simulink model "Arm_new_inv_kin"  (R2014b)
settings: Solver=ode45  StartTime=0.0  StopTime=1  RelTol=1e-3
libraries: mblibv1 x29
settings Model: Creator=Qizong  LastModifiedBy=Qizong
settings SimMechanicsCC: VisOnUpdateDiagram=on  VisDuringSimulation=on

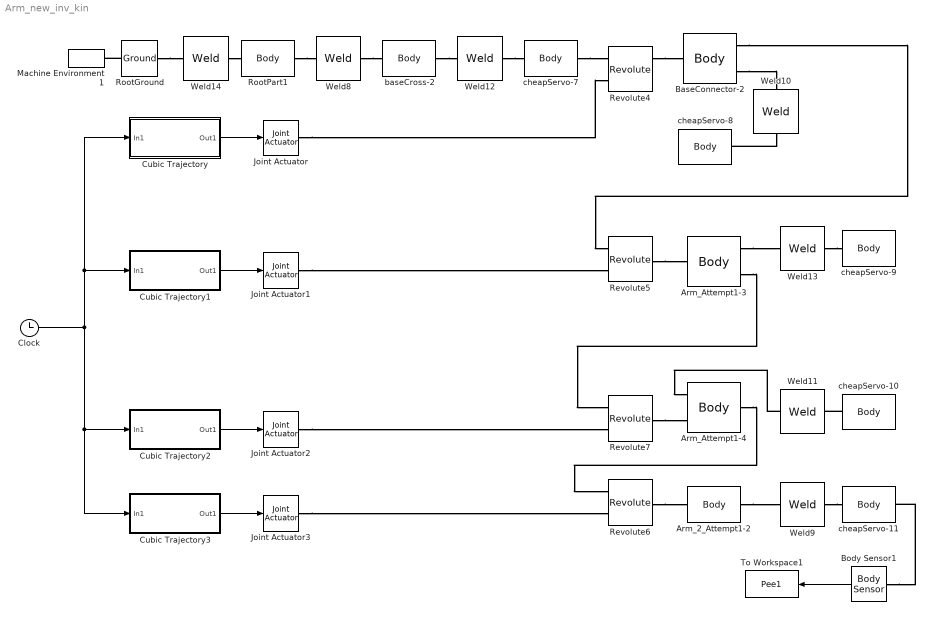
== system Arm_new_inv_kin ==
  Arm_2_Attempt1-2 : mblibv1/Bodies/Body  LConnTagsString=CS3  RConnTagsString=CS2  UpdateFromCAD=on  DialogClass=MechanicalBodyBlock  Mass=0.00482788  MassUnits=kg  InertiaUnits=kg*m^2  Inertia=[1.93456e-06,-1.28538e-09,1.03955e-07;-1.28538e-09,2.88684e-06,-1.81312e-09;1.03955e-07,-1.81312e-09,1.07e-06]  Shape=Cylinder  ShapeDims=[1 1]  ShapeUnits=m  ShapeUse=false  Density=1  DensityUnits=kg/m^3  DensityUse=false  GraphicsMode=GFXFILE  GraphicsFileName=Arm_new - Arm_2_Attempt1-1.STL  BodyColorSelMode=COLORPALETTE  BodyColor=[0.792157;0.819608;0.933333]  AttachedToCS=CS1  CG=Right$CG$[0.0802063 0.117359 0.26392]$WORLD$WORLD$m$[0 0 -1;0 1 0;1 0 0]$3x3 Transform$rad$WORLD$false$none  WorkingFrames=Right$CS1$[0.0387132 0.111386 0.303805]$WORLD$WORLD$m$[0 0 -1;0 1 0;1 0 0]$3x3 Transform$rad$WORLD$false$none#Right$CS2$[0.0387132 0.111386 0.303805]$WORLD$WORLD$m$[1 0 0;0 1 0;0 0 1]$3x3 Transform$rad$WORLD$true$none#Left$CS3$[0.0587132 0.117456 0.279]$WORLD$WORLD$m$[1 0 0;0 1 0;0 0 1]$3x3 Transform$rad$WORLD$true$none  CGPos=[0.0802063 0.117359 0.26392]  CGRot=[0 0 -1;0 1 0;1 0 0]  CS0Pos=[]  CS0Rot=[]  CS1Pos=[0.0387132 0.111386 0.303805]  CS1Rot=[0 0 -1;0 1 0;1 0 0]  CS2Pos=[0.0387132 0.111386 0.303805]  CS2Rot=[1 0 0;0 1 0;0 0 1]  CS3Pos=[0.0587132 0.117456 0.279]  CS3Rot=[1 0 0;0 1 0;0 0 1]  CS4Pos=[]  CS4Rot=[]  CS5Pos=[]  CS5Rot=[]  CS6Pos=[]  CS6Rot=[]  CS7Pos=[]  CS7Rot=[]  CS8Pos=[]  CS8Rot=[]  CS9Pos=[]  CS9Rot=[]  CS10Pos=[]  CS10Rot=[]  CS11Pos=[]  CS11Rot=[]  CS12Pos=[]  CS12Rot=[]  CS13Pos=[]  CS13Rot=[]  CS14Pos=[]  CS14Rot=[]  CS15Pos=[]  CS15Rot=[]  CS16Pos=[]  CS16Rot=[]  CS17Pos=[]  CS17Rot=[]  CS18Pos=[]  CS18Rot=[]  CS19Pos=[]  CS19Rot=[]  CS20Pos=[]  CS20Rot=[]
  Arm_Attempt1-3 : mblibv1/Bodies/Body  LConnTagsString=CS2  RConnTagsString=CS3|CS4  UpdateFromCAD=on  DialogClass=MechanicalBodyBlock  Mass=0.00663008  MassUnits=kg  InertiaUnits=kg*m^2  Inertia=[3.57587e-06,1.12045e-09,4.59326e-07;1.12045e-09,4.47292e-06,-5.09042e-09;4.59326e-07,-5.09042e-09,1.05685e-06]  Shape=Cylinder  ShapeDims=[1 1]  ShapeUnits=m  ShapeUse=false  Density=1  DensityUnits=kg/m^3  DensityUse=false  GraphicsMode=GFXFILE  GraphicsFileName=Arm_new - Arm_Attempt1-1.STL  BodyColorSelMode=COLORPALETTE  BodyColor=[0.792157;0.819608;0.933333]  AttachedToCS=CS1  CG=Right$CG$[0.0109911 0.0413075 0.267024]$WORLD$WORLD$m$[0 -1 0;0 0 -1;1 0 0]$3x3 Transform$rad$WORLD$false$none  WorkingFrames=Right$CS1$[0.0169693 -0.00863884 0.305399]$WORLD$WORLD$m$[0 -1 0;0 0 -1;1 0 0]$3x3 Transform$rad$WORLD$false$none#Left$CS2$[0.0108991 0.00236116 0.279]$WORLD$WORLD$m$[1 0 0;0 1 0;0 0 1]$3x3 Transform$rad$WORLD$true$none#Right$CS3$[0.00496925 0.0753612 0.277464]$WORLD$WORLD$m$[1 0 0;0 1 0;0 0 1]$3x3 Transform$rad$WORLD$true$none#Right$CS4$[0.0109693 0.0698112 0.279]$WORLD$WORLD$m$[1 0 0;0 1 0;0 0 1]$3x3 Transform$rad$WORLD$true$none  CGPos=[0.0109911 0.0413075 0.267024]  CGRot=[0 -1 0;0 0 -1;1 0 0]  CS0Pos=[]  CS0Rot=[]  CS1Pos=[0.0169693 -0.00863884 0.305399]  CS1Rot=[0 -1 0;0 0 -1;1 0 0]  CS2Pos=[0.0108991 0.00236116 0.279]  CS2Rot=[1 0 0;0 1 0;0 0 1]  CS3Pos=[0.00496925 0.0753612 0.277464]  CS3Rot=[1 0 0;0 1 0;0 0 1]  CS4Pos=[0.0109693 0.0698112 0.279]  CS4Rot=[1 0 0;0 1 0;0 0 1]  CS5Pos=[]  CS5Rot=[]  CS6Pos=[]  CS6Rot=[]  CS7Pos=[]  CS7Rot=[]  CS8Pos=[]  CS8Rot=[]  CS9Pos=[]  CS9Rot=[]  CS10Pos=[]  CS10Rot=[]  CS11Pos=[]  CS11Rot=[]  CS12Pos=[]  CS12Rot=[]  CS13Pos=[]  CS13Rot=[]  CS14Pos=[]  CS14Rot=[]  CS15Pos=[]  CS15Rot=[]  CS16Pos=[]  CS16Rot=[]  CS17Pos=[]  CS17Rot=[]  CS18Pos=[]  CS18Rot=[]  CS19Pos=[]  CS19Rot=[]  CS20Pos=[]  CS20Rot=[]
  Arm_Attempt1-4 : mblibv1/Bodies/Body  LConnTagsString=CS2|CS4  RConnTagsString=CS3  UpdateFromCAD=on  DialogClass=MechanicalBodyBlock  Mass=0.00663008  MassUnits=kg  InertiaUnits=kg*m^2  Inertia=[3.57587e-06,1.12045e-09,4.59326e-07;1.12045e-09,4.47292e-06,-5.09042e-09;4.59326e-07,-5.09042e-09,1.05685e-06]  Shape=Cylinder  ShapeDims=[1 1]  ShapeUnits=m  ShapeUse=false  Density=1  DensityUnits=kg/m^3  DensityUse=false  GraphicsMode=GFXFILE  GraphicsFileName=Arm_new - Arm_Attempt1-2.STL  BodyColorSelMode=COLORPALETTE  BodyColor=[0.792157;0.819608;0.933333]  AttachedToCS=CS1  CG=Right$CG$[0.0385735 0.0972853 0.267024]$WORLD$WORLD$m$[0 -0.707107 -0.707107;0 0.707107 -0.707107;1 0 0]$3x3 Transform$rad$WORLD$false$none  WorkingFrames=Right$CS1$[0.00748332 0.0577407 0.305399]$WORLD$WORLD$m$[0 -0.707107 -0.707107;0 0.707107 -0.707107;1 0 0]$3x3 Transform$rad$WORLD$false$none#Left$CS2$[0.0667389 0.117279 0.265014]$WORLD$WORLD$m$[1 0 0;0 1 0;0 0 1]$3x3 Transform$rad$WORLD$true$none#Right$CS3$[0.0587132 0.117456 0.279]$WORLD$WORLD$m$[1 0 0;0 1 0;0 0 1]$3x3 Transform$rad$WORLD$true$none#Left$CS4$[0.0109693 0.0698112 0.279]$WORLD$WORLD$m$[1 0 0;0 1 0;0 0 1]$3x3 Transform$rad$WORLD$true$none  CGPos=[0.0385735 0.0972853 0.267024]  CGRot=[0 -0.707107 -0.707107;0 0.707107 -0.707107;1 0 0]  CS0Pos=[]  CS0Rot=[]  CS1Pos=[0.00748332 0.0577407 0.305399]  CS1Rot=[0 -0.707107 -0.707107;0 0.707107 -0.707107;1 0 0]  CS2Pos=[0.0667389 0.117279 0.265014]  CS2Rot=[1 0 0;0 1 0;0 0 1]  CS3Pos=[0.0587132 0.117456 0.279]  CS3Rot=[1 0 0;0 1 0;0 0 1]  CS4Pos=[0.0109693 0.0698112 0.279]  CS4Rot=[1 0 0;0 1 0;0 0 1]  CS5Pos=[]  CS5Rot=[]  CS6Pos=[]  CS6Rot=[]  CS7Pos=[]  CS7Rot=[]  CS8Pos=[]  CS8Rot=[]  CS9Pos=[]  CS9Rot=[]  CS10Pos=[]  CS10Rot=[]  CS11Pos=[]  CS11Rot=[]  CS12Pos=[]  CS12Rot=[]  CS13Pos=[]  CS13Rot=[]  CS14Pos=[]  CS14Rot=[]  CS15Pos=[]  CS15Rot=[]  CS16Pos=[]  CS16Rot=[]  CS17Pos=[]  CS17Rot=[]  CS18Pos=[]  CS18Rot=[]  CS19Pos=[]  CS19Rot=[]  CS20Pos=[]  CS20Rot=[]
  BaseConnector-2 : mblibv1/Bodies/Body  LConnTagsString=CS2  RConnTagsString=CS3|CS4  UpdateFromCAD=on  DialogClass=MechanicalBodyBlock  Mass=0.00289161  MassUnits=kg  InertiaUnits=kg*m^2  Inertia=[1.81369e-07,-9.46923e-10,-2.62761e-09;-9.46923e-10,3.3813e-07,-2.11475e-08;-2.62761e-09,-2.11475e-08,2.75643e-07]  Shape=Cylinder  ShapeDims=[1 1]  ShapeUnits=m  ShapeUse=false  Density=1  DensityUnits=kg/m^3  DensityUse=false  GraphicsMode=GFXFILE  GraphicsFileName=Arm_new - BaseConnector-1.STL  BodyColorSelMode=COLORPALETTE  BodyColor=[1;1;1]  AttachedToCS=CS1  CG=Right$CG$[0.00564211 -0.00116004 0.271229]$WORLD$WORLD$m$[1 0 0;0 1 0;0 0 1]$3x3 Transform$rad$WORLD$false$none  WorkingFrames=Right$CS1$[0.00554911 -0.00353884 0.2601]$WORLD$WORLD$m$[1 0 0;0 1 0;0 0 1]$3x3 Transform$rad$WORLD$false$none#Left$CS2$[0.00554911 -0.00353884 0.27]$WORLD$WORLD$m$[1 0 0;0 1 0;0 0 1]$3x3 Transform$rad$WORLD$true$none#Right$CS3$[0.0108991 0.00236116 0.279]$WORLD$WORLD$m$[1 0 0;0 1 0;0 0 1]$3x3 Transform$rad$WORLD$true$none#Right$CS4$[0.00554911 -0.00353884 0.2601]$WORLD$WORLD$m$[1 0 0;0 1 0;0 0 1]$3x3 Transform$rad$WORLD$true$none  CGPos=[0.00564211 -0.00116004 0.271229]  CGRot=[1 0 0;0 1 0;0 0 1]  CS0Pos=[]  CS0Rot=[]  CS1Pos=[0.00554911 -0.00353884 0.2601]  CS1Rot=[1 0 0;0 1 0;0 0 1]  CS2Pos=[0.00554911 -0.00353884 0.27]  CS2Rot=[1 0 0;0 1 0;0 0 1]  CS3Pos=[0.0108991 0.00236116 0.279]  CS3Rot=[1 0 0;0 1 0;0 0 1]  CS4Pos=[0.00554911 -0.00353884 0.2601]  CS4Rot=[1 0 0;0 1 0;0 0 1]  CS5Pos=[]  CS5Rot=[]  CS6Pos=[]  CS6Rot=[]  CS7Pos=[]  CS7Rot=[]  CS8Pos=[]  CS8Rot=[]  CS9Pos=[]  CS9Rot=[]  CS10Pos=[]  CS10Rot=[]  CS11Pos=[]  CS11Rot=[]  CS12Pos=[]  CS12Rot=[]  CS13Pos=[]  CS13Rot=[]  CS14Pos=[]  CS14Rot=[]  CS15Pos=[]  CS15Rot=[]  CS16Pos=[]  CS16Rot=[]  CS17Pos=[]  CS17Rot=[]  CS18Pos=[]  CS18Rot=[]  CS19Pos=[]  CS19Rot=[]  CS20Pos=[]  CS20Rot=[]
  Body Sensor1 : mblibv1/Sensors &  Actuators/Body Sensor  UpdateFromCAD=off  PhysicalDomain=Mechanical  PortType=blob  Muxed=on  Pose=off  Angle=on  AngleUnits=deg  ArcVelocity=off  ArcVelocityUnits=deg/s  ArcAcceleration=off  ArcAccelerationUnits=deg/s^2  CoordPosition=on  CoordPositionUnits=m  Velocity=off  VelocityUnits=m/s  Acceleration=off  AccelerationUnits=m/s^2  Quaternion=on  QuaternionDT=off  QuaternionDDT=off  QuaternionUnits=off  OutputVector=[1]  ActiveIO=on  Width=3  DialogClass=MechanicalSensorBlock  ReferenceFrame=Absolute (World)
  Clock : Clock
  Cubic Trajectory : Subsystem  mask(Cubic Trajectory){}
  Cubic Trajectory1 : Subsystem  mask(Cubic Trajectory){}
  Cubic Trajectory2 : Subsystem  mask(Cubic Trajectory){}
  Cubic Trajectory3 : Subsystem  mask(Cubic Trajectory){}
  Joint Actuator{,1..3} (4 alike) : mblibv1/Sensors &  Actuators/Joint Actuator  UpdateFromCAD=off  PhysicalDomain=Mechanical  PortType=blob  ActuationStyle=Motion  AngleUnits=rad  ArcVelocityUnits=rad/s  ArcAccelerationUnits=rad/s^2  CoordPositionUnits=m  VelocityUnits=m/s  AccelerationUnits=m/s^2  ForceUnits=N  TorqueUnits=N*m  ActiveIO=on  Width=3  DialogClass=MechanicalActuatorBlock  Primitive=R1  ReferenceFrame=Absolute (World)
  Machine Environment1 : mblibv1/Bodies/Machine Environment  PortType=env  PhysicalDomain=Mechanical  DialogTemplateClass=MECH.MachineEnvironment  SyncWhenCopied=off  Gravity=[0 -9.81 0]  GravityUnits=m/s^2  GravityAsSignal=off  Dimensionality=Auto-detect  AnalysisType=Forward dynamics  LinearAssemblyTolerance=1e-3  LinearAssemblyToleranceUnits=m  AngularAssemblyTolerance=1e-3  AngularAssemblyToleranceUnits=rad  ConstraintSolverType=Stabilizing  ConstraintRelTolerance=1e-4  ConstraintAbsTolerance=1e-4  UseRobustSingularityHandling=off  RedundancyAnalysisToleranceType=Automatically select tolerance  RedundancyAnalysisTolerance=1e-14  StatePerturbationType=Fixed  PerturbationSize=1e-5  VisualizeMachine=on  BodyVisualizationType=Use model default body geometries  BodyColorSelMode=Use model default  DefaultBodyColor=[1 0 0]
  Revolute4 : mblibv1/Joints/Revolute  LConnTagsString=__newl0|SA1  RConnTagsString=__newr0|SA1  UpdateFromCAD=on  NumSAPorts=2  CutJoint=off  MarkAsCut=off  Primitives=prismatic  PrimitiveProps=R1$World$[0,1,0]$revolute  DialogClass=JointBlock  R1Axis=[0,1,0]
  Revolute5 : mblibv1/Joints/Revolute  LConnTagsString=__newl0|SA1  RConnTagsString=__newr0  UpdateFromCAD=on  NumSAPorts=1  CutJoint=off  MarkAsCut=off  Primitives=prismatic  PrimitiveProps=R1$World$[0,0,-1]$revolute  DialogClass=JointBlock  R1Axis=[0,0,-1]
  Revolute6 : mblibv1/Joints/Revolute  LConnTagsString=__newl0|SA1  RConnTagsString=__newr0  UpdateFromCAD=on  NumSAPorts=1  CutJoint=off  MarkAsCut=off  Primitives=prismatic  PrimitiveProps=R1$World$[0,0,-1]$revolute  DialogClass=JointBlock  R1Axis=[0,0,-1]
  Revolute7 : mblibv1/Joints/Revolute  LConnTagsString=__newl0|SA1  RConnTagsString=__newr0  UpdateFromCAD=on  NumSAPorts=1  CutJoint=off  MarkAsCut=off  Primitives=prismatic  PrimitiveProps=R1$World$[0,0,-1]$revolute  DialogClass=JointBlock  R1Axis=[0,0,-1]
  RootGround : mblibv1/Bodies/Ground  UpdateFromCAD=on  LeftPortType=env  RightPortType=workingframe  PhysicalDomain=Mechanical  DialogClass=GroundBlock  CoordPosition=[0.024952,0.026403,0.267905]  CoordPositionUnits=m  StateVectorMgrId=2  MachineId=[1 0]  ShowEnvPort=on  ParameterChecksum=[449264359, 1693856497, 1829625602, 1228565225]  TopologyChecksum=[1919634279, 3543996490, 3153834687, 3124392432]
  RootPart1 : mblibv1/Bodies/Body  LConnTagsString=CS3  RConnTagsString=CS2  UpdateFromCAD=on  DialogClass=MechanicalBodyBlock  Mass=0  MassUnits=kg  InertiaUnits=kg*m^2  Inertia=[0,0,0;0,0,0;0,0,0]  Shape=Cylinder  ShapeDims=[1 1]  ShapeUnits=m  ShapeUse=false  Density=1  DensityUnits=kg/m^3  DensityUse=false  GraphicsMode=MACHINE_DEFAULT  BodyColorSelMode=MACHINE_DEFAULT  BodyColor=[1;0;0]  AttachedToCS=CS1  CG=Right$CG$[0.024952 0.026403 0.267905]$WORLD$WORLD$m$[1 0 0;0 1 0;0 0 1]$3x3 Transform$rad$WORLD$false$none  WorkingFrames=Right$CS1$[0 0 0]$WORLD$WORLD$m$[1 0 0;0 1 0;0 0 1]$3x3 Transform$rad$WORLD$false$none#Right$CS2$[0.00554913 -0.0339934 0.27051]$WORLD$WORLD$m$[1 0 0;0 1 0;0 0 1]$3x3 Transform$rad$WORLD$true$none#Left$CS3$[0.024952 0.026403 0.267905]$WORLD$WORLD$m$[1 0 0;0 1 0;0 0 1]$3x3 Transform$rad$WORLD$true$none  CGPos=[0.024952 0.026403 0.267905]  CGRot=[1 0 0;0 1 0;0 0 1]  CS0Pos=[]  CS0Rot=[]  CS1Pos=[0 0 0]  CS1Rot=[1 0 0;0 1 0;0 0 1]  CS2Pos=[0.00554913 -0.0339934 0.27051]  CS2Rot=[1 0 0;0 1 0;0 0 1]  CS3Pos=[0.024952 0.026403 0.267905]  CS3Rot=[1 0 0;0 1 0;0 0 1]  CS4Pos=[]  CS4Rot=[]  CS5Pos=[]  CS5Rot=[]  CS6Pos=[]  CS6Rot=[]  CS7Pos=[]  CS7Rot=[]  CS8Pos=[]  CS8Rot=[]  CS9Pos=[]  CS9Rot=[]  CS10Pos=[]  CS10Rot=[]  CS11Pos=[]  CS11Rot=[]  CS12Pos=[]  CS12Rot=[]  CS13Pos=[]  CS13Rot=[]  CS14Pos=[]  CS14Rot=[]  CS15Pos=[]  CS15Rot=[]  CS16Pos=[]  CS16Rot=[]  CS17Pos=[]  CS17Rot=[]  CS18Pos=[]  CS18Rot=[]  CS19Pos=[]  CS19Rot=[]  CS20Pos=[]  CS20Rot=[]
  To Workspace1 : ToWorkspace  VariableName=Pee1  SaveFormat=Timeseries  SampleTime=-1
  Weld{8..14} (7 alike) : mblibv1/Joints/Weld  LConnTagsString=__newl0  RConnTagsString=__newr0  UpdateFromCAD=on  NumSAPorts=0  CutJoint=off  MarkAsCut=off  Primitives=weld  PrimitiveProps=W$WORLD$[0.57735,0.57735,0.57735]$weld  DialogClass=JointBlock  WAxis=[0.57735,0.57735,0.57735]
  baseCross-2 : mblibv1/Bodies/Body  LConnTagsString=CS2  RConnTagsString=CS3  UpdateFromCAD=on  DialogClass=MechanicalBodyBlock  Mass=0.0338588  MassUnits=kg  InertiaUnits=kg*m^2  Inertia=[9.50419e-05,-4.72341e-14,1.07796e-10;-4.72341e-14,0.000189164,-1.55231e-07;1.07796e-10,-1.55231e-07,9.48987e-05]  Shape=Cylinder  ShapeDims=[1 1]  ShapeUnits=m  ShapeUse=false  Density=1  DensityUnits=kg/m^3  DensityUse=false  GraphicsMode=GFXFILE  GraphicsFileName=Arm_new - baseCross-1.STL  BodyColorSelMode=COLORPALETTE  BodyColor=[1;1;1]  AttachedToCS=CS1  CG=Right$CG$[0.00554913 -0.0339934 0.27051]$WORLD$WORLD$m$[1 0 0;0 1 0;0 0 1]$3x3 Transform$rad$WORLD$false$none  WorkingFrames=Right$CS1$[0.00554911 -0.0334388 0.27]$WORLD$WORLD$m$[1 0 0;0 1 0;0 0 1]$3x3 Transform$rad$WORLD$false$none#Left$CS2$[0.00554913 -0.0339934 0.27051]$WORLD$WORLD$m$[1 0 0;0 1 0;0 0 1]$3x3 Transform$rad$WORLD$true$none#Right$CS3$[-0.000350892 -0.0175388 0.27]$WORLD$WORLD$m$[1 0 0;0 1 0;0 0 1]$3x3 Transform$rad$WORLD$true$none  CGPos=[0.00554913 -0.0339934 0.27051]  CGRot=[1 0 0;0 1 0;0 0 1]  CS0Pos=[]  CS0Rot=[]  CS1Pos=[0.00554911 -0.0334388 0.27]  CS1Rot=[1 0 0;0 1 0;0 0 1]  CS2Pos=[0.00554913 -0.0339934 0.27051]  CS2Rot=[1 0 0;0 1 0;0 0 1]  CS3Pos=[-0.000350892 -0.0175388 0.27]  CS3Rot=[1 0 0;0 1 0;0 0 1]  CS4Pos=[]  CS4Rot=[]  CS5Pos=[]  CS5Rot=[]  CS6Pos=[]  CS6Rot=[]  CS7Pos=[]  CS7Rot=[]  CS8Pos=[]  CS8Rot=[]  CS9Pos=[]  CS9Rot=[]  CS10Pos=[]  CS10Rot=[]  CS11Pos=[]  CS11Rot=[]  CS12Pos=[]  CS12Rot=[]  CS13Pos=[]  CS13Rot=[]  CS14Pos=[]  CS14Rot=[]  CS15Pos=[]  CS15Rot=[]  CS16Pos=[]  CS16Rot=[]  CS17Pos=[]  CS17Rot=[]  CS18Pos=[]  CS18Rot=[]  CS19Pos=[]  CS19Rot=[]  CS20Pos=[]  CS20Rot=[]
  cheapServo-10 : mblibv1/Bodies/Body  RConnTagsString=CS2  UpdateFromCAD=on  DialogClass=MechanicalBodyBlock  Mass=0.00769542  MassUnits=kg  InertiaUnits=kg*m^2  Inertia=[4.96531e-07,3.23519e-08,0;3.23519e-08,4.44048e-07,0;0,0,7.67618e-07]  Shape=Cylinder  ShapeDims=[1 1]  ShapeUnits=m  ShapeUse=false  Density=1  DensityUnits=kg/m^3  DensityUse=false  GraphicsMode=GFXFILE  GraphicsFileName=Arm_new - cheapServo-5.STL  BodyColorSelMode=COLORPALETTE  BodyColor=[0.494118;0.494118;0.494118]  AttachedToCS=CS1  CG=Right$CG$[0.0548517 0.113736 0.263624]$WORLD$WORLD$m$[-0.707107 0 0.707107;-0.707107 0 -0.707107;0 -1 0]$3x3 Transform$rad$WORLD$false$none  WorkingFrames=Right$CS1$[0.054612 0.113496 0.265014]$WORLD$WORLD$m$[-0.707107 0 0.707107;-0.707107 0 -0.707107;0 -1 0]$3x3 Transform$rad$WORLD$false$none#Right$CS2$[0.0667389 0.117279 0.265014]$WORLD$WORLD$m$[1 0 0;0 1 0;0 0 1]$3x3 Transform$rad$WORLD$true$none  CGPos=[0.0548517 0.113736 0.263624]  CGRot=[-0.707107 0 0.707107;-0.707107 0 -0.707107;0 -1 0]  CS0Pos=[]  CS0Rot=[]  CS1Pos=[0.054612 0.113496 0.265014]  CS1Rot=[-0.707107 0 0.707107;-0.707107 0 -0.707107;0 -1 0]  CS2Pos=[0.0667389 0.117279 0.265014]  CS2Rot=[1 0 0;0 1 0;0 0 1]  CS3Pos=[]  CS3Rot=[]  CS4Pos=[]  CS4Rot=[]  CS5Pos=[]  CS5Rot=[]  CS6Pos=[]  CS6Rot=[]  CS7Pos=[]  CS7Rot=[]  CS8Pos=[]  CS8Rot=[]  CS9Pos=[]  CS9Rot=[]  CS10Pos=[]  CS10Rot=[]  CS11Pos=[]  CS11Rot=[]  CS12Pos=[]  CS12Rot=[]  CS13Pos=[]  CS13Rot=[]  CS14Pos=[]  CS14Rot=[]  CS15Pos=[]  CS15Rot=[]  CS16Pos=[]  CS16Rot=[]  CS17Pos=[]  CS17Rot=[]  CS18Pos=[]  CS18Rot=[]  CS19Pos=[]  CS19Rot=[]  CS20Pos=[]  CS20Rot=[]
  cheapServo-11 : mblibv1/Bodies/Body  LConnTagsString=CS2  RConnTagsString=CS1  UpdateFromCAD=on  DialogClass=MechanicalBodyBlock  Mass=0.00769542  MassUnits=kg  InertiaUnits=kg*m^2  Inertia=[4.96531e-07,3.23519e-08,0;3.23519e-08,4.44048e-07,0;0,0,7.67618e-07]  Shape=Cylinder  ShapeDims=[1 1]  ShapeUnits=m  ShapeUse=false  Density=1  DensityUnits=kg/m^3  DensityUse=false  GraphicsMode=GFXFILE  GraphicsFileName=Arm_new - cheapServo-6.STL  BodyColorSelMode=COLORPALETTE  BodyColor=[0.49412 0.49412 0.49412]  AttachedToCS=CS1  CG=Right$CG$[0.105855 0.117286 0.265314]$WORLD$WORLD$m$[0 1 0;0 0 1;1 0 0]$3x3 Transform$rad$WORLD$false$none  WorkingFrames=Right$CS1$[0.104465 0.117286 0.265653]$World$World$m$[0 1 0;0 0 1;1 0 0]$3x3 Transform$rad$WORLD$true$none#Left$CS2$[0.0387132 0.111386 0.303805]$WORLD$WORLD$m$[1 0 0;0 1 0;0 0 1]$3x3 Transform$rad$WORLD$true$none  CGPos=[0.105855 0.117286 0.265314]  CGRot=[0 1 0;0 0 1;1 0 0]  CS0Pos=[]  CS0Rot=[]  CS1Pos=[0.104465 0.117286 0.265653]  CS1Rot=[0 1 0;0 0 1;1 0 0]  CS2Pos=[0.0387132 0.111386 0.303805]  CS2Rot=[1 0 0;0 1 0;0 0 1]  CS3Pos=[]  CS3Rot=[]  CS4Pos=[]  CS4Rot=[]  CS5Pos=[]  CS5Rot=[]  CS6Pos=[]  CS6Rot=[]  CS7Pos=[]  CS7Rot=[]  CS8Pos=[]  CS8Rot=[]  CS9Pos=[]  CS9Rot=[]  CS10Pos=[]  CS10Rot=[]  CS11Pos=[]  CS11Rot=[]  CS12Pos=[]  CS12Rot=[]  CS13Pos=[]  CS13Rot=[]  CS14Pos=[]  CS14Rot=[]  CS15Pos=[]  CS15Rot=[]  CS16Pos=[]  CS16Rot=[]  CS17Pos=[]  CS17Rot=[]  CS18Pos=[]  CS18Rot=[]  CS19Pos=[]  CS19Rot=[]  CS20Pos=[]  CS20Rot=[]
  cheapServo-7 : mblibv1/Bodies/Body  LConnTagsString=CS3  RConnTagsString=CS2  UpdateFromCAD=on  DialogClass=MechanicalBodyBlock  Mass=0.00769542  MassUnits=kg  InertiaUnits=kg*m^2  Inertia=[4.96531e-07,3.23519e-08,0;3.23519e-08,4.44048e-07,0;0,0,7.67618e-07]  Shape=Cylinder  ShapeDims=[1 1]  ShapeUnits=m  ShapeUse=false  Density=1  DensityUnits=kg/m^3  DensityUse=false  GraphicsMode=GFXFILE  GraphicsFileName=Arm_new - cheapServo-1.STL  BodyColorSelMode=COLORPALETTE  BodyColor=[0.494118;0.494118;0.494118]  AttachedToCS=CS1  CG=Right$CG$[0.00554911 -0.0206986 0.275011]$WORLD$WORLD$m$[0 0 -1;0 1 0;1 0 0]$3x3 Transform$rad$WORLD$false$none  WorkingFrames=Right$CS1$[0.00554911 -0.0220888 0.27535]$WORLD$WORLD$m$[0 0 -1;0 1 0;1 0 0]$3x3 Transform$rad$WORLD$false$none#Right$CS2$[0.00554911 -0.00353884 0.27]$WORLD$WORLD$m$[1 0 0;0 1 0;0 0 1]$3x3 Transform$rad$WORLD$true$none#Left$CS3$[-0.000350892 -0.0175388 0.27]$WORLD$WORLD$m$[1 0 0;0 1 0;0 0 1]$3x3 Transform$rad$WORLD$true$none  CGPos=[0.00554911 -0.0206986 0.275011]  CGRot=[0 0 -1;0 1 0;1 0 0]  CS0Pos=[]  CS0Rot=[]  CS1Pos=[0.00554911 -0.0220888 0.27535]  CS1Rot=[0 0 -1;0 1 0;1 0 0]  CS2Pos=[0.00554911 -0.00353884 0.27]  CS2Rot=[1 0 0;0 1 0;0 0 1]  CS3Pos=[-0.000350892 -0.0175388 0.27]  CS3Rot=[1 0 0;0 1 0;0 0 1]  CS4Pos=[]  CS4Rot=[]  CS5Pos=[]  CS5Rot=[]  CS6Pos=[]  CS6Rot=[]  CS7Pos=[]  CS7Rot=[]  CS8Pos=[]  CS8Rot=[]  CS9Pos=[]  CS9Rot=[]  CS10Pos=[]  CS10Rot=[]  CS11Pos=[]  CS11Rot=[]  CS12Pos=[]  CS12Rot=[]  CS13Pos=[]  CS13Rot=[]  CS14Pos=[]  CS14Rot=[]  CS15Pos=[]  CS15Rot=[]  CS16Pos=[]  CS16Rot=[]  CS17Pos=[]  CS17Rot=[]  CS18Pos=[]  CS18Rot=[]  CS19Pos=[]  CS19Rot=[]  CS20Pos=[]  CS20Rot=[]
  cheapServo-8 : mblibv1/Bodies/Body  LConnTagsString=CS2  UpdateFromCAD=on  DialogClass=MechanicalBodyBlock  Mass=0.00769542  MassUnits=kg  InertiaUnits=kg*m^2  Inertia=[4.96531e-07,3.23519e-08,0;3.23519e-08,4.44048e-07,0;0,0,7.67618e-07]  Shape=Cylinder  ShapeDims=[1 1]  ShapeUnits=m  ShapeUse=false  Density=1  DensityUnits=kg/m^3  DensityUse=false  GraphicsMode=GFXFILE  GraphicsFileName=Arm_new - cheapServo-2.STL  BodyColorSelMode=COLORPALETTE  BodyColor=[0.494118;0.494118;0.494118]  AttachedToCS=CS1  CG=Right$CG$[0.00588816 0.00236116 0.26326]$WORLD$WORLD$m$[-1 0 0;0 0 -1;0 -1 0]$3x3 Transform$rad$WORLD$false$none  WorkingFrames=Right$CS1$[0.00554911 0.00236116 0.26465]$WORLD$WORLD$m$[-1 0 0;0 0 -1;0 -1 0]$3x3 Transform$rad$WORLD$false$none#Left$CS2$[0.00554911 -0.00353884 0.2601]$WORLD$WORLD$m$[1 0 0;0 1 0;0 0 1]$3x3 Transform$rad$WORLD$true$none  CGPos=[0.00588816 0.00236116 0.26326]  CGRot=[-1 0 0;0 0 -1;0 -1 0]  CS0Pos=[]  CS0Rot=[]  CS1Pos=[0.00554911 0.00236116 0.26465]  CS1Rot=[-1 0 0;0 0 -1;0 -1 0]  CS2Pos=[0.00554911 -0.00353884 0.2601]  CS2Rot=[1 0 0;0 1 0;0 0 1]  CS3Pos=[]  CS3Rot=[]  CS4Pos=[]  CS4Rot=[]  CS5Pos=[]  CS5Rot=[]  CS6Pos=[]  CS6Rot=[]  CS7Pos=[]  CS7Rot=[]  CS8Pos=[]  CS8Rot=[]  CS9Pos=[]  CS9Rot=[]  CS10Pos=[]  CS10Rot=[]  CS11Pos=[]  CS11Rot=[]  CS12Pos=[]  CS12Rot=[]  CS13Pos=[]  CS13Rot=[]  CS14Pos=[]  CS14Rot=[]  CS15Pos=[]  CS15Rot=[]  CS16Pos=[]  CS16Rot=[]  CS17Pos=[]  CS17Rot=[]  CS18Pos=[]  CS18Rot=[]  CS19Pos=[]  CS19Rot=[]  CS20Pos=[]  CS20Rot=[]
  cheapServo-9 : mblibv1/Bodies/Body  LConnTagsString=CS2  UpdateFromCAD=on  DialogClass=MechanicalBodyBlock  Mass=0.00769542  MassUnits=kg  InertiaUnits=kg*m^2  Inertia=[4.96531e-07,3.23519e-08,0;3.23519e-08,4.44048e-07,0;0,0,7.67618e-07]  Shape=Cylinder  ShapeDims=[1 1]  ShapeUnits=m  ShapeUse=false  Density=1  DensityUnits=kg/m^3  DensityUse=false  GraphicsMode=GFXFILE  GraphicsFileName=Arm_new - cheapServo-3.STL  BodyColorSelMode=COLORPALETTE  BodyColor=[0.494118;0.494118;0.494118]  AttachedToCS=CS1  CG=Right$CG$[0.0108693 0.0644502 0.263624]$WORLD$WORLD$m$[0 0 1;-1 0 0;0 -1 0]$3x3 Transform$rad$WORLD$false$none  WorkingFrames=Right$CS1$[0.0108693 0.0641112 0.265014]$WORLD$WORLD$m$[0 0 1;-1 0 0;0 -1 0]$3x3 Transform$rad$WORLD$false$none#Left$CS2$[0.00496925 0.0753612 0.277464]$WORLD$WORLD$m$[1 0 0;0 1 0;0 0 1]$3x3 Transform$rad$WORLD$true$none  CGPos=[0.0108693 0.0644502 0.263624]  CGRot=[0 0 1;-1 0 0;0 -1 0]  CS0Pos=[]  CS0Rot=[]  CS1Pos=[0.0108693 0.0641112 0.265014]  CS1Rot=[0 0 1;-1 0 0;0 -1 0]  CS2Pos=[0.00496925 0.0753612 0.277464]  CS2Rot=[1 0 0;0 1 0;0 0 1]  CS3Pos=[]  CS3Rot=[]  CS4Pos=[]  CS4Rot=[]  CS5Pos=[]  CS5Rot=[]  CS6Pos=[]  CS6Rot=[]  CS7Pos=[]  CS7Rot=[]  CS8Pos=[]  CS8Rot=[]  CS9Pos=[]  CS9Rot=[]  CS10Pos=[]  CS10Rot=[]  CS11Pos=[]  CS11Rot=[]  CS12Pos=[]  CS12Rot=[]  CS13Pos=[]  CS13Rot=[]  CS14Pos=[]  CS14Rot=[]  CS15Pos=[]  CS15Rot=[]  CS16Pos=[]  CS16Rot=[]  CS17Pos=[]  CS17Rot=[]  CS18Pos=[]  CS18Rot=[]  CS19Pos=[]  CS19Rot=[]  CS20Pos=[]  CS20Rot=[]
  wires:
  Cubic Trajectory/1(Out1) -> Joint Actuator/1
  Cubic Trajectory1/1(Out1) -> Joint Actuator1/1
  Cubic Trajectory2/1(Out1) -> Joint Actuator2/1
  Cubic Trajectory3/1(Out1) -> Joint Actuator3/1
  Clock/1 -> Cubic Trajectory/1(In1), Cubic Trajectory1/1(In1), Cubic Trajectory3/1(In1), Cubic Trajectory2/1(In1)
  Body Sensor1/1 -> To Workspace1/1
  connections:
  Arm_2_Attempt1-2/RConn1 -- Weld9/LConn1
  BaseConnector-2/RConn2 -- Weld10/LConn1
  RootGround/RConn1 -- Weld14/LConn1
  Weld9/RConn1 -- cheapServo-11/LConn1
  Weld11/RConn1 -- Arm_Attempt1-4/LConn1
  Arm_Attempt1-3/RConn2 -- Revolute7/LConn1
  Revolute5/RConn1 -- Arm_Attempt1-3/LConn1
  Revolute6/RConn1 -- Arm_2_Attempt1-2/LConn1
  Arm_Attempt1-3/RConn1 -- Weld13/LConn1
  baseCross-2/RConn1 -- Weld12/LConn1
  cheapServo-7/RConn1 -- Revolute4/LConn1
  Weld12/RConn1 -- cheapServo-7/LConn1
  Body Sensor1/LConn1 -- cheapServo-11/RConn1
  Revolute4/RConn1 -- BaseConnector-2/LConn1
  Weld10/RConn1 -- cheapServo-8/LConn1
  cheapServo-10/RConn1 -- Weld11/LConn1
  Arm_Attempt1-4/RConn1 -- Revolute6/LConn1
  Weld8/RConn1 -- baseCross-2/LConn1
  RootGround/LConn1 -- Machine Environment1/RConn1
  RootPart1/RConn1 -- Weld8/LConn1
  Weld13/RConn1 -- cheapServo-9/LConn1
  BaseConnector-2/RConn1 -- Revolute5/LConn1
  Weld14/RConn1 -- RootPart1/LConn1
  Revolute7/RConn1 -- Arm_Attempt1-4/LConn2
  Joint Actuator/RConn1 -- Revolute4/LConn2
  Joint Actuator1/RConn1 -- Revolute5/LConn2
  Joint Actuator2/RConn1 -- Revolute7/LConn2
  Joint Actuator3/RConn1 -- Revolute6/LConn2

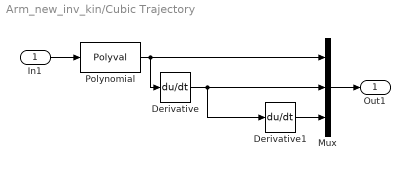
== system Arm_new_inv_kin/Cubic Trajectory ==
  In1 : Inport
  Derivative : Derivative
  Derivative1 : Derivative
  Mux : Mux  Inputs=3
  Polynomial : Polyval  Coefs=|
      | [-1.5608
      |     2.3462
      |          0
      |          0]
  Out1 : Outport
  wires:
  Mux/1 -> Out1/1
  Derivative/1 -> Derivative1/1, Mux/2
  Derivative1/1 -> Mux/3
  In1/1 -> Polynomial/1
  Polynomial/1 -> Derivative/1, Mux/1

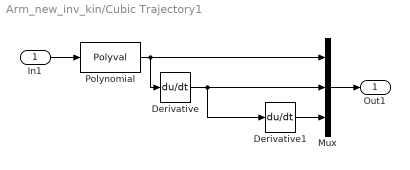
== system Arm_new_inv_kin/Cubic Trajectory1 ==
  In1 : Inport
  Derivative : Derivative
  Derivative1 : Derivative
  Mux : Mux  Inputs=3
  Polynomial : Polyval  Coefs=|
      | [ 0.0100
      |    -0.0100
      |          0
      |          0]
  Out1 : Outport
  wires:
  Polynomial/1 -> Mux/1, Derivative/1
  In1/1 -> Polynomial/1
  Derivative1/1 -> Mux/3
  Derivative/1 -> Mux/2, Derivative1/1
  Mux/1 -> Out1/1

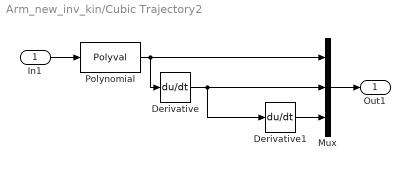
== system Arm_new_inv_kin/Cubic Trajectory2 ==
  In1 : Inport
  Derivative : Derivative
  Derivative1 : Derivative
  Mux : Mux  Inputs=3
  Polynomial : Polyval  Coefs=|
      | [-2.0319
      |     3.0529
      |          0
      |          0]
  Out1 : Outport
  wires:
  Mux/1 -> Out1/1
  Derivative/1 -> Derivative1/1, Mux/2
  Derivative1/1 -> Mux/3
  In1/1 -> Polynomial/1
  Polynomial/1 -> Derivative/1, Mux/1

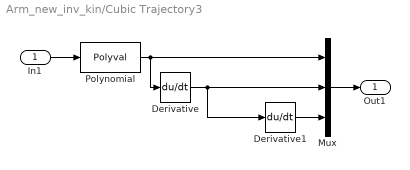
== system Arm_new_inv_kin/Cubic Trajectory3 ==
  In1 : Inport
  Derivative : Derivative
  Derivative1 : Derivative
  Mux : Mux  Inputs=3
  Polynomial : Polyval  Coefs=|
      | [-0.6180
      |     0.9320
      |          0
      |          0]
  Out1 : Outport
  wires:
  Polynomial/1 -> Mux/1, Derivative/1
  In1/1 -> Polynomial/1
  Derivative1/1 -> Mux/3
  Derivative/1 -> Mux/2, Derivative1/1
  Mux/1 -> Out1/1
